simulink model "lab14_exercise"  (R2015b)
settings: Solver=VariableStepAuto  StartTime=0.0  StopTime=10.0  RelTol=1e-3
settings Model: Creator=MAHEEN  LastModifiedBy=MAHEEN

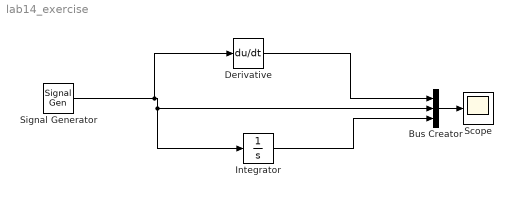
== system lab14_exercise ==
  Bus Creator : BusCreator  Inputs=3
  Derivative : Derivative
  Integrator : Integrator  InitialCondition=-1
  Scope : Scope
  Signal Generator : SignalGenerator  WaveForm=square  Units=rad/sec
  wires:
  Signal Generator/1 -> Bus Creator/2, Integrator/1, Derivative/1
  Derivative/1 -> Bus Creator/1
  Integrator/1 -> Bus Creator/3
  Bus Creator/1 -> Scope/1
